simulink model "mpptfixed0312"  (R2024b)
settings: Solver=VariableStepAuto  StartTime=0.0  StopTime=0.1  RelTol=1e-3
libraries: spsDiodeLib x4, spsPVArrayLib x3, spsSeriesRLCBranchLib x2, spsCurrentMeasurementLib x1, spsDCVoltageSourceLib x1, spsGroundLib x1, spsMosfetLib x1, spsVoltageMeasurementLib x1, sps_lib x1
settings Model: Creator=psybe  LastModifiedBy=psybe

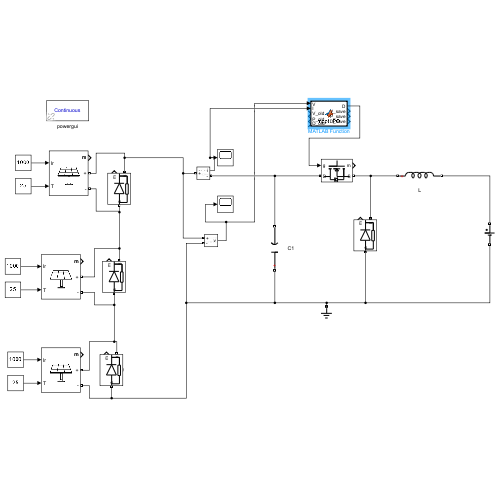
[thumbnail: Simulink's stored preview of the top-level diagram]
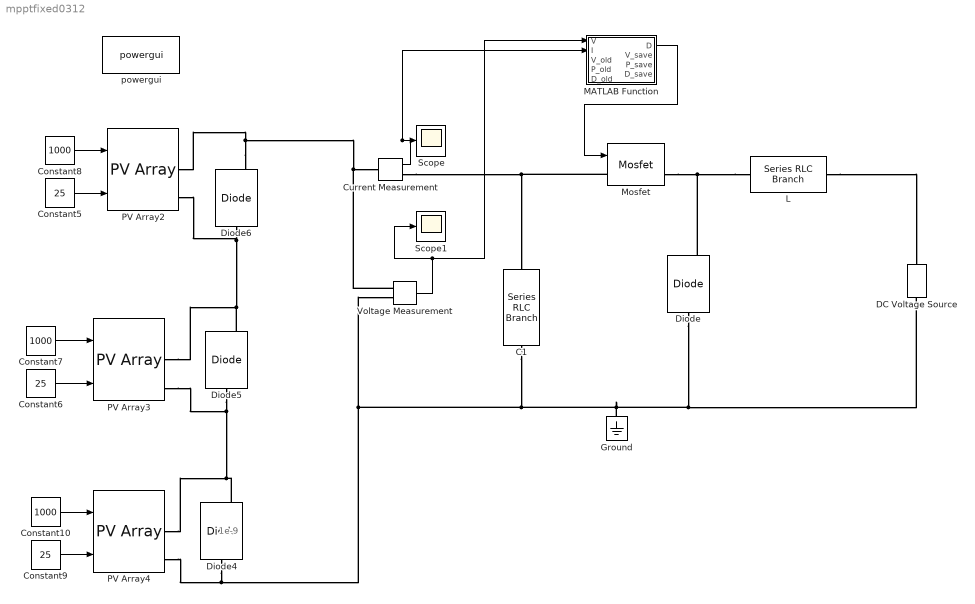
== system mpptfixed0312 ==
  note: 1e-9
  C1 : spsSeriesRLCBranchLib/Series RLC Branch  LConnTagsString=__new0  RConnTagsString=__new0  BranchType=C  Resistance=1e-3  Inductance=1e-3  SetiL0=off  InitialCurrent=0  Capacitance=100e-6  Setx0=on  InitialVoltage=49  Measurements=None
  Constant10 : Constant  Value=1000
  Constant5 : Constant  Value=25
  Constant6 : Constant  Value=25
  Constant7 : Constant  Value=1000
  Constant8 : Constant  Value=1000
  Constant9 : Constant  Value=25
  Current Measurement : spsCurrentMeasurementLib/Current Measurement  PhasorSimulation=off  OutputType=Complex  PSBequivalent=0
  DC Voltage Source : spsDCVoltageSourceLib/DC Voltage Source  Amplitude=48  Measurements=None
  Diode : spsDiodeLib/Diode  Ron=0.001  Lon=0  Vf=0.8  IC=0  UseSnubber=0  Rs=500  Cs=250e-9  Measurements=on
  Diode4 : spsDiodeLib/Diode  Ron=0.001  Lon=0  Vf=0.8  IC=0  UseSnubber=0  Rs=500  Cs=1e-9  Measurements=on
  Diode5 : spsDiodeLib/Diode  Ron=0.001  Lon=0  Vf=0.8  IC=0  UseSnubber=0  Rs=500  Cs=1e-9  Measurements=on
  Diode6 : spsDiodeLib/Diode  Ron=0.001  Lon=0  Vf=0.8  IC=0  UseSnubber=0  Rs=500  Cs=1e-9  Measurements=on
  Ground : spsGroundLib/Ground  LConnTagsString=a
  L : spsSeriesRLCBranchLib/Series RLC Branch  LConnTagsString=__new0  RConnTagsString=__new0  BranchType=L  Resistance=1  Inductance=10e-6  SetiL0=off  InitialCurrent=0  Capacitance=1e-6  Setx0=off  InitialVoltage=0  Measurements=None
  MATLAB Function : MATLAB Function  TreatAsAtomicUnit=on
  Mosfet : spsMosfetLib/Mosfet  Ron=0.1  Lon=0  Rd=0.01  Vfd=0  IC=0  Rs=1e5  Cs=inf  Measurements=on
  PV Array2 : spsPVArrayLib/PV Array  Npar=1  Nser=1  PlotType=array @ 1000 W/m2 & specified temperatures  S_vec="[ 1000  500  100 ]"  Temp_C_vec="[ 45 25  ]"  ModuleName=User-defined  PlotWhenSelected=off  Pm=213.15  Ncell=60  Voc=36.3  Isc=7.84  Vm=29  Im=7.35  beta_Voc_pc=-0.36099  alpha_Isc_pc=0.102  beta_Voc=-0.13104  alpha_Isc=0.0079968  IL=7.8654  I0=2.9273e-10  nI=0.98119  Rsh=313.0553  Rs=0.39381  RobustModel=off  RobustCellTemperature=313.3991  BAL=on  Tc=1e-6  Tfilter=5e-5
  PV Array3 : spsPVArrayLib/PV Array  Npar=1  Nser=1  PlotType=array @ 1000 W/m2 & specified temperatures  S_vec="[ 1000  500  100 ]"  Temp_C_vec="[ 45 25  ]"  ModuleName=User-defined  PlotWhenSelected=off  Pm=213.15  Ncell=60  Voc=36.3  Isc=7.84  Vm=29  Im=7.35  beta_Voc_pc=-0.36099  alpha_Isc_pc=0.102  beta_Voc=-0.13104  alpha_Isc=0.0079968  IL=7.8654  I0=2.9273e-10  nI=0.98119  Rsh=313.0553  Rs=0.39381  RobustModel=off  RobustCellTemperature=313.3991  BAL=on  Tc=1e-6  Tfilter=5e-5
  PV Array4 : spsPVArrayLib/PV Array  Npar=1  Nser=1  PlotType=array @ 1000 W/m2 & specified temperatures  S_vec="[ 1000  500  100 ]"  Temp_C_vec="[ 45 25  ]"  ModuleName=User-defined  PlotWhenSelected=off  Pm=213.15  Ncell=60  Voc=36.3  Isc=7.84  Vm=29  Im=7.35  beta_Voc_pc=-0.36099  alpha_Isc_pc=0.102  beta_Voc=-0.13104  alpha_Isc=0.0079968  IL=7.8654  I0=2.9273e-10  nI=0.98119  Rsh=313.0553  Rs=0.39381  RobustModel=off  RobustCellTemperature=313.3991  BAL=on  Tc=1e-6  Tfilter=5e-5
  Scope : Scope
  Scope1 : Scope
  Voltage Measurement : spsVoltageMeasurementLib/Voltage Measurement  PhasorSimulation=off  OutputType=Complex  PSBequivalent=0
  powergui : sps_lib/powergui  Priority=1  SimulationMode=Continuous  SampleTime=1e-6  frequency=60  Iterations=50  frequencyindice=0  Pbase=100e6  ErrMax=1e-4  UnitsV=kV  UnitsW=MW  buscounter=0  FunctionMessages=off  echomessages=off  EnableUseOfTLC=off  CurrentSourceSwitches=off  DisableSnubberDevices=off  DisableRonSwitches=off  DisableVfSwitches=off  DisplayEquations=off  AutomaticDiscreteSolvers=off  SolverType=Tustin/Backward Euler (TBE)  Interpol=off  ExternalGateDelay=off  methode=off  Ts=100  x0status=blocks  SPID=on  SwTol=0  HookPort=off  NonlinearTolerance=1e-4  nMaxIteration=100  ContinueOnMaxIteration=off  RestoreLinks=warning  ResistiveCurrentMeasurement=off  Frange=[0:2:500]  Ylog=off  Xlog=on  ShowGrid=off  save=off  variable=ZData  structure=0  ZoomFFT=off  StartTime=0.0  cycles=1  DisplayStyle=1  fundamental=60  FreqAxis=off  MaxFrequency=1000  frequencyindicesteady=1  RmsSteady=1  display=off
  wires:
  MATLAB Function/1(D) -> Mosfet/1
  Current Measurement/1 -> MATLAB Function/2(I), Scope/1
  Voltage Measurement/1 -> MATLAB Function/1(V), Scope1/1
  Constant9/1 -> PV Array4/2
  Constant10/1 -> PV Array4/1
  Constant6/1 -> PV Array3/2
  Constant8/1 -> PV Array2/1
  Constant7/1 -> PV Array3/1
  Constant5/1 -> PV Array2/2
  connections:
  Diode4/LConn1 -- Voltage Measurement/LConn2 -- C1/LConn1 -- Ground/LConn1 -- Diode/LConn1 -- DC Voltage Source/LConn1 -- PV Array4/RConn2
  Mosfet/LConn1 -- Current Measurement/RConn1 -- C1/RConn1
  Diode6/RConn1 -- Voltage Measurement/LConn1 -- Current Measurement/LConn1 -- PV Array2/RConn1
  L/LConn1 -- Mosfet/RConn1 -- Diode/RConn1
  L/RConn1 -- DC Voltage Source/RConn1
  Diode6/LConn1 -- PV Array2/RConn2 -- PV Array3/RConn1 -- Diode5/RConn1
  Diode5/LConn1 -- PV Array3/RConn2 -- PV Array4/RConn1 -- Diode4/RConn1

== matlab function mpptfixed0312/MATLAB Function ==
  data: V input; D output; I input; V_old input; P_old input; D_old input; V_save output; P_save output; D_save output
function [D, V_save, P_save, D_save] = mppt_PO(V, I, V_old, P_old, D_old)
% P&O MPPT Algorithm - 초기 튐 개선 버전

delta_D = 0.005;
D_init  = 0.5;      % 초기 듀티비 (50%)
V_min   = 1.0;      % 유효 전압 최소값 (노이즈 필터)
settle_threshold = 0.01; % 정착 판별용

P = V * I;

% ── 초기화 조건 ──────────────────────────────────────────
% V가 너무 낮으면 아직 PV가 기동 안 된 것 → 듀티 고정
if V < V_min
    D      = D_init;
    V_save = V_old;   % 이전 값 유지
    P_save = P_old;
    D_save = D_old;
    return;           % 함수 즉시 종료
end

% 최초 호출 (모든 이전값이 0)
if V_old == 0 && P_old == 0 && D_old == 0
    D      = D_init;
    V_save = V;
    P_save = P;
    D_save = D;
    return;
end

% ── P&O 로직 ─────────────────────────────────────────────
dP = P - P_old;
dV = V - V_old;

% 변화량이 노이즈 수준이면 듀티 유지 (불필요한 진동 방지)
if abs(dP) < settle_threshold && abs(dV) < settle_threshold
    D = D_old;
else
    if dP > 0
        if dV > 0
            D = D_old - delta_D;
        else
            D = D_old + delta_D;
        end
    else
        if dV > 0
            D = D_old + delta_D;
        else
            D = D_old - delta_D;
        end
    end
end

% ── 듀티비 클램핑 ────────────────────────────────────────
D = max(0.1, min(0.9, D));

% ── 출력 저장 ────────────────────────────────────────────
V_save = V;
P_save = P;
D_save = D;

end
